simulink model "Template_v4_1_0_2024b_Jetson"  (R2024b)
settings: Solver=ode4  StartTime=0.0  StopTime=tsim  FixedStep=baseRate  RelTol=1e-6  AbsTol=1e-6
undefined symbols (not defined in the file): a1, a2, a3, b0, b1, b2, b3, baseRate, dataRate, DiscIntNeverNeededParam, drop_states_ARM, drop_states_BLACK, drop_states_BLUE, drop_states_RED, F_red_X_nominal, F_red_Y_nominal, F_thrusters_BLACK, F_thrusters_BLUE, F_thrusters_RED, Gamma1_el, Gamma1_sh, Gamma1_wr, Gamma2_el, Gamma2_sh, Gamma2_wr, Gamma3_el, Gamma3_sh, Gamma3_wr, Gamma4_el, Gamma4_sh, Gamma4_wr, Gamma5_el, Gamma5_sh, Gamma5_wr, Gamma6_el, Gamma6_sh, Gamma6_wr, home_states_BLACK, home_states_BLUE, home_states_RED, IBLACK, IBLUE, IDIST, IEE, init_states_BLACK, init_states_BLUE, init_states_RED, IPROX, IRED, K_BLACK, K_BLUE, K_RED, Kd_elarm, Kd_sharm, Kd_tb, Kd_tblue, Kd_tr, Kd_wrarm, Kd_xb, Kd_xblue ... (+45)
libraries: simulink x30, nvidiaSharedBlocks x19, MainLibrary x6, dspinverses x3, nvidiaIMUSensorslib x1
(part 6 of 8)

== system Template_v4_1_0_2024b_Jetson/1 - Experiment Logic/Phase #3: Experiment/Sub-Phase #3 /Desired Position BLUE/Wrap ==
  In1 : Inport
  Atan2 : Trigonometry  Operator=atan2
  Cos : Trigonometry  Operator=cos
  Sin : Trigonometry
  Out1 : Outport
  wires:
  In1/1 -> Sin/1, Cos/1
  Cos/1 -> Atan2/2
  Atan2/1 -> Out1/1
  Sin/1 -> Atan2/1

== system Template_v4_1_0_2024b_Jetson/1 - Experiment Logic/Phase #3: Experiment/Sub-Phase #3 /Desired Position RED/Calculate Circular Tracking ==
  Angular Frequency : Inport
  Constant1 : Constant  Value=xLength/2
  Constant2 : Constant  Value=yLength/2
  Cos : Trigonometry  Operator=cos
  Gain : Gain  Gain=0.85
  Gain1 : Gain  Gain=0.85
  Sin : Trigonometry
  Sum1 : Sum  Inputs=|++
  Sum2 : Sum  Inputs=|++
  Target X : Outport
  Target Y : Outport  Port=2
  wires:
  Constant2/1 -> Sum2/2
  Angular Frequency/1 -> Sin/1, Cos/1
  Constant1/1 -> Sum1/2
  Cos/1 -> Gain/1
  Gain1/1 -> Sum2/1
  Sin/1 -> Gain1/1
  Gain/1 -> Sum1/1
  Sum2/1 -> Target Y/1
  Sum1/1 -> Target X/1

== system Template_v4_1_0_2024b_Jetson/1 - Experiment Logic/Phase #3: Experiment/Sub-Phase #3 /Desired Position RED/Calculate Time since Phase #3 Start ==
  Constant2 : Constant  Value=Phase2_End  SampleTime=-1
  Subsystem : Subsystem
  Subtract3 : Sum  Inputs=+-
  Time : Outport  VectorParamsAs1DForOutWhenUnconnected=off
  wires:
  Subtract3/1 -> Time/1
  Constant2/1 -> Subtract3/2
  Subsystem/1(Time) -> Subtract3/1

== system Template_v4_1_0_2024b_Jetson/1 - Experiment Logic/Phase #3: Experiment/Sub-Phase #3 /Desired Position RED/Wrap ==
  In1 : Inport
  Atan2 : Trigonometry  Operator=atan2
  Cos : Trigonometry  Operator=cos
  Sin : Trigonometry
  Out1 : Outport
  wires:
  In1/1 -> Sin/1, Cos/1
  Cos/1 -> Atan2/2
  Atan2/1 -> Out1/1
  Sin/1 -> Atan2/1

== system Template_v4_1_0_2024b_Jetson/1 - Experiment Logic/Phase #3: Experiment/Sub-Phase #4/Desired Position BLACK/BLACK_Rz Desired ==
  Desired Rate (BLACK) : Constant  Value=0.03490659  SampleTime=-1
  Product : Product
  Subsystem : Subsystem
  Rz_Target : Outport  VectorParamsAs1DForOutWhenUnconnected=off
  wires:
  Product/1 -> Rz_Target/1
  Desired Rate (BLACK)/1 -> Product/1
  Subsystem/1(Time) -> Product/2

== system Template_v4_1_0_2024b_Jetson/1 - Experiment Logic/Phase #3: Experiment/Sub-Phase #4/Desired Position BLACK/Wrap ==
  In1 : Inport
  Atan2 : Trigonometry  Operator=atan2
  Cos : Trigonometry  Operator=cos
  Sin : Trigonometry
  Out1 : Outport
  wires:
  In1/1 -> Sin/1, Cos/1
  Cos/1 -> Atan2/2
  Atan2/1 -> Out1/1
  Sin/1 -> Atan2/1

== system Template_v4_1_0_2024b_Jetson/1 - Experiment Logic/Phase #3: Experiment/Sub-Phase #4/Desired Position BLUE/Calculate Circular Tracking ==
  Angular Frequency : Inport
  Constant1 : Constant  Value=xLength/2
  Constant2 : Constant  Value=yLength/2
  Cos : Trigonometry  Operator=cos
  Gain : Gain  Gain=-0.85
  Gain1 : Gain  Gain=-0.85
  Sin : Trigonometry
  Sum1 : Sum  Inputs=|++
  Sum2 : Sum  Inputs=|++
  Target X : Outport
  Target Y : Outport  Port=2
  wires:
  Constant2/1 -> Sum2/2
  Angular Frequency/1 -> Sin/1, Cos/1
  Constant1/1 -> Sum1/2
  Cos/1 -> Gain/1
  Gain1/1 -> Sum2/1
  Sin/1 -> Gain1/1
  Gain/1 -> Sum1/1
  Sum2/1 -> Target Y/1
  Sum1/1 -> Target X/1

== system Template_v4_1_0_2024b_Jetson/1 - Experiment Logic/Phase #3: Experiment/Sub-Phase #4/Desired Position BLUE/Calculate Time since Phase #3 Start ==
  Constant2 : Constant  Value=Phase2_End  SampleTime=-1
  Subsystem : Subsystem
  Subtract3 : Sum  Inputs=+-
  Time : Outport  VectorParamsAs1DForOutWhenUnconnected=off
  wires:
  Subtract3/1 -> Time/1
  Constant2/1 -> Subtract3/2
  Subsystem/1(Time) -> Subtract3/1

== system Template_v4_1_0_2024b_Jetson/1 - Experiment Logic/Phase #3: Experiment/Sub-Phase #4/Desired Position BLUE/Wrap ==
  In1 : Inport
  Atan2 : Trigonometry  Operator=atan2
  Cos : Trigonometry  Operator=cos
  Sin : Trigonometry
  Out1 : Outport
  wires:
  In1/1 -> Sin/1, Cos/1
  Cos/1 -> Atan2/2
  Atan2/1 -> Out1/1
  Sin/1 -> Atan2/1

== system Template_v4_1_0_2024b_Jetson/1 - Experiment Logic/Phase #3: Experiment/Sub-Phase #4/Desired Position RED/Calculate Circular Tracking ==
  Angular Frequency : Inport
  Constant1 : Constant  Value=xLength/2
  Constant2 : Constant  Value=yLength/2
  Cos : Trigonometry  Operator=cos
  Gain : Gain  Gain=0.85
  Gain1 : Gain  Gain=0.85
  Sin : Trigonometry
  Sum1 : Sum  Inputs=|++
  Sum2 : Sum  Inputs=|++
  Target X : Outport
  Target Y : Outport  Port=2
  wires:
  Constant2/1 -> Sum2/2
  Angular Frequency/1 -> Sin/1, Cos/1
  Constant1/1 -> Sum1/2
  Cos/1 -> Gain/1
  Gain1/1 -> Sum2/1
  Sin/1 -> Gain1/1
  Gain/1 -> Sum1/1
  Sum2/1 -> Target Y/1
  Sum1/1 -> Target X/1

== system Template_v4_1_0_2024b_Jetson/1 - Experiment Logic/Phase #3: Experiment/Sub-Phase #4/Desired Position RED/Calculate Time since Phase #3 Start ==
  Constant2 : Constant  Value=Phase2_End  SampleTime=-1
  Subsystem : Subsystem
  Subtract3 : Sum  Inputs=+-
  Time : Outport  VectorParamsAs1DForOutWhenUnconnected=off
  wires:
  Subtract3/1 -> Time/1
  Constant2/1 -> Subtract3/2
  Subsystem/1(Time) -> Subtract3/1

== system Template_v4_1_0_2024b_Jetson/1 - Experiment Logic/Phase #3: Experiment/Sub-Phase #4/Desired Position RED/Wrap ==
  In1 : Inport
  Atan2 : Trigonometry  Operator=atan2
  Cos : Trigonometry  Operator=cos
  Sin : Trigonometry
  Out1 : Outport
  wires:
  In1/1 -> Sin/1, Cos/1
  Cos/1 -> Atan2/2
  Atan2/1 -> Out1/1
  Sin/1 -> Atan2/1

== system Template_v4_1_0_2024b_Jetson/PhaseSpace Camera Code/Use Hardware to Obtain States/Receive and Process Phasespace Data/Check for Sychronization (Updated)/Enabled Subsystem2 ==
  In1 : Inport
  Enable : EnablePort
  Universal Time : Outport
  wires:
  In1/1 -> Universal Time/1

== system Template_v4_1_0_2024b_Jetson/PhaseSpace Camera Code/Use Hardware to Obtain States/Receive and Process Phasespace Data/Check for Sychronization (Updated)/Send Sync. Time ==
  Universal Time : Inport
  Change BLACK Behavior : Subsystem  TreatAsAtomicUnit=on
  Change BLUE Behavior : Subsystem  TreatAsAtomicUnit=on
  Change RED Behavior : Subsystem  TreatAsAtomicUnit=on
  Data Store Read : DataStoreRead  DataStoreName=WhoAmI  IndexOptions=Index vector (dialog)  Indices=1  OutputSizes=1
  Data Store Read2 : DataStoreRead  DataStoreName=isSim  IndexOptions=Index vector (dialog)  Indices=1  OutputSizes=1
  This IF block determines whether or not to run the BLACK sim/exp : If  NumInputs=2  IfExpression=u1 == 2 & u2 == 0  ShowElse=off
  This IF block determines whether or not to run the BLUE sim/exp : If  NumInputs=2  IfExpression=u1 == 3 & u2 == 0  ShowElse=off
  "This IF block determines whether or not to run the RED sim/exp " : If  NumInputs=2  IfExpression=u1 == 1 & u2 == 0  ShowElse=off
  wires:
  Data Store Read/1 -> This IF block determines whether or not to run the BLUE sim/exp/1, This IF block determines whether or not to run the BLACK sim/exp/1, "This IF block determines whether or not to run the RED sim/exp "/1
  This IF block determines whether or not to run the BLUE sim/exp/1 -> Change BLUE Behavior/Action
  "This IF block determines whether or not to run the RED sim/exp "/1 -> Change RED Behavior/Action
  Data Store Read2/1 -> This IF block determines whether or not to run the BLACK sim/exp/2, This IF block determines whether or not to run the BLUE sim/exp/2, "This IF block determines whether or not to run the RED sim/exp "/2
  This IF block determines whether or not to run the BLACK sim/exp/1 -> Change BLACK Behavior/Action
  Universal Time/1 -> Change BLACK Behavior/1(Universal Time), Change RED Behavior/1(Universal Time), Change BLUE Behavior/1(Universal Time)

== system Template_v4_1_0_2024b_Jetson/PhaseSpace Camera Code/Use Hardware to Obtain States/Store BLACK Data/Calculate True Time Step/Enabled Subsystem3 ==
  y2-y1 : Inport
  Enable : EnablePort
  dy(t)/dt : Outport
  wires:
  y2-y1/1 -> dy(t)/dt/1

== system Template_v4_1_0_2024b_Jetson/PhaseSpace Camera Code/Use Hardware to Obtain States/Store BLACK Data/Subsystem1/Enabled Subsystem ==
  y : Inport
  dt : Inport  Port=2
  Enable : EnablePort
  Constant2 : Constant  Value=0.1
  Delay : Delay  DelayLength=1
  MATLAB Function : MATLAB Function  TreatAsAtomicUnit=on
  dy/dt : Outport
  wires:
  Constant2/1 -> MATLAB Function/3(tau)
  dt/1 -> MATLAB Function/2(dt)
  Delay/1 -> MATLAB Function/4(ema_prev)
  MATLAB Function/2(ema) -> Delay/1
  y/1 -> MATLAB Function/1(y)
  MATLAB Function/1(dy) -> dy/dt/1

== system Template_v4_1_0_2024b_Jetson/PhaseSpace Camera Code/Use Hardware to Obtain States/Store BLACK Data/Subsystem2/Enabled Subsystem ==
  y : Inport
  dt : Inport  Port=2
  Enable : EnablePort
  Constant2 : Constant  Value=0.1
  Delay : Delay  DelayLength=1
  MATLAB Function : MATLAB Function  TreatAsAtomicUnit=on
  dy/dt : Outport
  wires:
  Constant2/1 -> MATLAB Function/3(tau)
  dt/1 -> MATLAB Function/2(dt)
  Delay/1 -> MATLAB Function/4(ema_prev)
  MATLAB Function/2(ema) -> Delay/1
  y/1 -> MATLAB Function/1(y)
  MATLAB Function/1(dy) -> dy/dt/1

== system Template_v4_1_0_2024b_Jetson/PhaseSpace Camera Code/Use Hardware to Obtain States/Store BLUE Data/Calculate True Time Step/Enabled Subsystem3 ==
  y2-y1 : Inport
  Enable : EnablePort
  dy(t)/dt : Outport
  wires:
  y2-y1/1 -> dy(t)/dt/1

== system Template_v4_1_0_2024b_Jetson/PhaseSpace Camera Code/Use Hardware to Obtain States/Store BLUE Data/Subsystem1/Enabled Subsystem ==
  y : Inport
  dt : Inport  Port=2
  Enable : EnablePort
  Constant2 : Constant  Value=0.1
  Delay : Delay  DelayLength=1
  MATLAB Function : MATLAB Function  TreatAsAtomicUnit=on
  dy/dt : Outport
  wires:
  Constant2/1 -> MATLAB Function/3(tau)
  dt/1 -> MATLAB Function/2(dt)
  Delay/1 -> MATLAB Function/4(ema_prev)
  MATLAB Function/2(ema) -> Delay/1
  y/1 -> MATLAB Function/1(y)
  MATLAB Function/1(dy) -> dy/dt/1

== system Template_v4_1_0_2024b_Jetson/PhaseSpace Camera Code/Use Hardware to Obtain States/Store BLUE Data/Subsystem2/Enabled Subsystem ==
  y : Inport
  dt : Inport  Port=2
  Enable : EnablePort
  Constant2 : Constant  Value=0.1
  Delay : Delay  DelayLength=1
  MATLAB Function : MATLAB Function  TreatAsAtomicUnit=on
  dy/dt : Outport
  wires:
  Constant2/1 -> MATLAB Function/3(tau)
  dt/1 -> MATLAB Function/2(dt)
  Delay/1 -> MATLAB Function/4(ema_prev)
  MATLAB Function/2(ema) -> Delay/1
  y/1 -> MATLAB Function/1(y)
  MATLAB Function/1(dy) -> dy/dt/1

== system Template_v4_1_0_2024b_Jetson/PhaseSpace Camera Code/Use Hardware to Obtain States/Store RED Data/Calculate True Time Step/Enabled Subsystem3 ==
  y2-y1 : Inport
  Enable : EnablePort
  dy(t)/dt : Outport
  wires:
  y2-y1/1 -> dy(t)/dt/1

== system Template_v4_1_0_2024b_Jetson/PhaseSpace Camera Code/Use Hardware to Obtain States/Store RED Data/Subsystem1/Enabled Subsystem ==
  y : Inport
  dt : Inport  Port=2
  Enable : EnablePort
  Constant2 : Constant  Value=0.1
  Delay : Delay  DelayLength=1
  MATLAB Function : MATLAB Function  TreatAsAtomicUnit=on
  dy/dt : Outport
  wires:
  Constant2/1 -> MATLAB Function/3(tau)
  dt/1 -> MATLAB Function/2(dt)
  Delay/1 -> MATLAB Function/4(ema_prev)
  MATLAB Function/2(ema) -> Delay/1
  y/1 -> MATLAB Function/1(y)
  MATLAB Function/1(dy) -> dy/dt/1

== system Template_v4_1_0_2024b_Jetson/PhaseSpace Camera Code/Use Hardware to Obtain States/Store RED Data/Subsystem2/Enabled Subsystem ==
  y : Inport
  dt : Inport  Port=2
  Enable : EnablePort
  Constant2 : Constant  Value=0.1
  Delay : Delay  DelayLength=1
  MATLAB Function : MATLAB Function  TreatAsAtomicUnit=on
  dy/dt : Outport
  wires:
  Constant2/1 -> MATLAB Function/3(tau)
  dt/1 -> MATLAB Function/2(dt)
  Delay/1 -> MATLAB Function/4(ema_prev)
  MATLAB Function/2(ema) -> Delay/1
  y/1 -> MATLAB Function/1(y)
  MATLAB Function/1(dy) -> dy/dt/1

== system Template_v4_1_0_2024b_Jetson/Simulate Plant Dynamics/BLACK Dynamics/Calculated & Store Measured States/Subsystem1/Enabled Subsystem ==
  y : Inport
  dt : Inport  Port=2
  Enable : EnablePort
  Constant2 : Constant  Value=0.1
  Delay : Delay  DelayLength=1
  MATLAB Function : MATLAB Function  TreatAsAtomicUnit=on
  dy/dt : Outport
  wires:
  Constant2/1 -> MATLAB Function/3(tau)
  dt/1 -> MATLAB Function/2(dt)
  Delay/1 -> MATLAB Function/4(ema_prev)
  MATLAB Function/2(ema) -> Delay/1
  y/1 -> MATLAB Function/1(y)
  MATLAB Function/1(dy) -> dy/dt/1

== system Template_v4_1_0_2024b_Jetson/Simulate Plant Dynamics/BLACK Dynamics/Calculated & Store Measured States/Subsystem2/Enabled Subsystem ==
  y : Inport
  dt : Inport  Port=2
  Enable : EnablePort
  Constant2 : Constant  Value=0.1
  Delay : Delay  DelayLength=1
  MATLAB Function : MATLAB Function  TreatAsAtomicUnit=on
  dy/dt : Outport
  wires:
  Constant2/1 -> MATLAB Function/3(tau)
  dt/1 -> MATLAB Function/2(dt)
  Delay/1 -> MATLAB Function/4(ema_prev)
  MATLAB Function/2(ema) -> Delay/1
  y/1 -> MATLAB Function/1(y)
  MATLAB Function/1(dy) -> dy/dt/1

== system Template_v4_1_0_2024b_Jetson/Simulate Plant Dynamics/BLACK Dynamics/Data @ Measurement Rate/Calculate True Time Step/Enabled Subsystem3 ==
  y2-y1 : Inport
  Enable : EnablePort
  dy(t)/dt : Outport
  wires:
  y2-y1/1 -> dy(t)/dt/1

== system Template_v4_1_0_2024b_Jetson/Simulate Plant Dynamics/BLUE Dynamics/Calculated & Store Measured States/Subsystem1/Enabled Subsystem ==
  y : Inport
  dt : Inport  Port=2
  Enable : EnablePort
  Constant2 : Constant  Value=0.1
  Delay : Delay  DelayLength=1
  MATLAB Function : MATLAB Function  TreatAsAtomicUnit=on
  dy/dt : Outport
  wires:
  Constant2/1 -> MATLAB Function/3(tau)
  dt/1 -> MATLAB Function/2(dt)
  Delay/1 -> MATLAB Function/4(ema_prev)
  MATLAB Function/2(ema) -> Delay/1
  y/1 -> MATLAB Function/1(y)
  MATLAB Function/1(dy) -> dy/dt/1

== system Template_v4_1_0_2024b_Jetson/Simulate Plant Dynamics/BLUE Dynamics/Calculated & Store Measured States/Subsystem2/Enabled Subsystem ==
  y : Inport
  dt : Inport  Port=2
  Enable : EnablePort
  Constant2 : Constant  Value=0.1
  Delay : Delay  DelayLength=1
  MATLAB Function : MATLAB Function  TreatAsAtomicUnit=on
  dy/dt : Outport
  wires:
  Constant2/1 -> MATLAB Function/3(tau)
  dt/1 -> MATLAB Function/2(dt)
  Delay/1 -> MATLAB Function/4(ema_prev)
  MATLAB Function/2(ema) -> Delay/1
  y/1 -> MATLAB Function/1(y)
  MATLAB Function/1(dy) -> dy/dt/1

== system Template_v4_1_0_2024b_Jetson/Simulate Plant Dynamics/BLUE Dynamics/Data @ Measurement Rate/Calculate True Time Step/Enabled Subsystem3 ==
  y2-y1 : Inport
  Enable : EnablePort
  dy(t)/dt : Outport
  wires:
  y2-y1/1 -> dy(t)/dt/1

== system Template_v4_1_0_2024b_Jetson/Simulate Plant Dynamics/RED and ARM Dynamics/RED + ARM/Calculated & Store Measured States/Subsystem3 ==
  dt : Inport
  y : Inport  Port=2
  Constant3 : Constant  Value=0
  Delay1 : Delay  DelayLength=1
  Enabled Subsystem : Subsystem  TreatAsAtomicUnit=on
  Relational Operator : RelationalOperator  Operator=~=  OutDataTypeStr=boolean  RndMeth=Simplest  InputSameDT=off
  Subtract1 : Sum  Inputs=+-
  dy/dt : Outport
  wires:
  Constant3/1 -> Relational Operator/2
  Relational Operator/1 -> Enabled Subsystem/Enable
  Delay1/1 -> Subtract1/2
  dt/1 -> Enabled Subsystem/2(dt)
  Subtract1/1 -> Relational Operator/1
  Enabled Subsystem/1(dy/dt) -> dy/dt/1
  y/1 -> Enabled Subsystem/1(y), Delay1/1, Subtract1/1

== system Template_v4_1_0_2024b_Jetson/Simulate Plant Dynamics/RED and ARM Dynamics/RED + ARM/Calculated & Store Measured States/Subsystem4 ==
  dt : Inport
  y : Inport  Port=2
  Constant3 : Constant  Value=0
  Delay1 : Delay  DelayLength=1
  Enabled Subsystem : Subsystem  TreatAsAtomicUnit=on
  Relational Operator : RelationalOperator  Operator=~=  OutDataTypeStr=boolean  RndMeth=Simplest  InputSameDT=off
  Subtract1 : Sum  Inputs=+-
  dy/dt : Outport
  wires:
  Constant3/1 -> Relational Operator/2
  Relational Operator/1 -> Enabled Subsystem/Enable
  Delay1/1 -> Subtract1/2
  dt/1 -> Enabled Subsystem/2(dt)
  Subtract1/1 -> Relational Operator/1
  Enabled Subsystem/1(dy/dt) -> dy/dt/1
  y/1 -> Enabled Subsystem/1(y), Delay1/1, Subtract1/1

== system Template_v4_1_0_2024b_Jetson/Simulate Plant Dynamics/RED and ARM Dynamics/RED + ARM/Calculated & Store Measured States/Subsystem5 ==
  dt : Inport
  y : Inport  Port=2
  Constant3 : Constant  Value=0
  Delay1 : Delay  DelayLength=1
  Enabled Subsystem : Subsystem  TreatAsAtomicUnit=on
  Relational Operator : RelationalOperator  Operator=~=  OutDataTypeStr=boolean  RndMeth=Simplest  InputSameDT=off
  Subtract1 : Sum  Inputs=+-
  dy/dt : Outport
  wires:
  Constant3/1 -> Relational Operator/2
  Relational Operator/1 -> Enabled Subsystem/Enable
  Delay1/1 -> Subtract1/2
  dt/1 -> Enabled Subsystem/2(dt)
  Subtract1/1 -> Relational Operator/1
  Enabled Subsystem/1(dy/dt) -> dy/dt/1
  y/1 -> Enabled Subsystem/1(y), Delay1/1, Subtract1/1

== system Template_v4_1_0_2024b_Jetson/Simulate Plant Dynamics/RED and ARM Dynamics/RED + ARM/Calculated & Store Measured States/Wrap ==
  Unwrapped Angle : Inport
  Atan2 : Trigonometry  Operator=atan2
  Cos : Trigonometry  Operator=cos
  Sin : Trigonometry
  Wrapped Angle : Outport
  wires:
  Unwrapped Angle/1 -> Sin/1, Cos/1
  Cos/1 -> Atan2/2
  Atan2/1 -> Wrapped Angle/1
  Sin/1 -> Atan2/1

== system Template_v4_1_0_2024b_Jetson/Simulate Plant Dynamics/RED and ARM Dynamics/RED + ARM/Calculated & Store True States/Wrap ==
  Unwrapped Angle : Inport
  Atan2 : Trigonometry  Operator=atan2
  Cos : Trigonometry  Operator=cos
  Sin : Trigonometry
  Wrapped Angle : Outport
  wires:
  Unwrapped Angle/1 -> Sin/1, Cos/1
  Cos/1 -> Atan2/2
  Atan2/1 -> Wrapped Angle/1
  Sin/1 -> Atan2/1

== system Template_v4_1_0_2024b_Jetson/Simulate Plant Dynamics/RED and ARM Dynamics/RED + ARM/Data @ Measurement Rate/Calculate True Time Step ==
  Data : Inport
  Time : Inport  Port=2
  Rate : Inport  Port=3
  Constant3 : Constant  Value=0
  Delay1 : Delay  DelayLength=1  InitialCondition=0
  Delay2 : Delay  DelayLength=1  InitialCondition=0
  Demux : Demux  Outputs=[1,5]
  Enabled Subsystem3 : Subsystem  TreatAsAtomicUnit=on
  MATLAB Function : MATLAB Function  TreatAsAtomicUnit=on
  Relational Operator : RelationalOperator  Operator=~=  OutDataTypeStr=boolean  RndMeth=Simplest  InputSameDT=off
  Subtract1 : Sum  Inputs=+-
  Subtract2 : Sum  Inputs=+-
  Terminator : Terminator
  dt_out : Outport
  wires:
  Rate/1 -> MATLAB Function/2(dataRate)
  MATLAB Function/1(dt_out) -> dt_out/1
  Time/1 -> Delay2/1, Subtract1/1
  Enabled Subsystem3/1(dy(t)/dt) -> MATLAB Function/1(dt)
  Data/1 -> Demux/1
  Subtract2/1 -> Relational Operator/1
  Relational Operator/1 -> Enabled Subsystem3/Enable
  Constant3/1 -> Relational Operator/2
  Demux/1 -> Subtract2/1, Delay1/1
  Delay1/1 -> Subtract2/2
  Demux/2 -> Terminator/1
  Subtract1/1 -> Enabled Subsystem3/1(y2-y1)
  Delay2/1 -> Subtract1/2

== system Template_v4_1_0_2024b_Jetson/Simulate Plant Dynamics/RED and ARM Dynamics/RED + ARM/Data @ Measurement Rate/Enabled Subsystem ==
  In1 : Inport
  Enable : EnablePort
  Out1 : Outport
  wires:
  In1/1 -> Out1/1

== system Template_v4_1_0_2024b_Jetson/Simulate Plant Dynamics/RED and ARM Dynamics/RED + ARM/Data @ Measurement Rate/Enabled Subsystem1 ==
  ThrustPer_Final : Inport
  Enable : EnablePort
  Out1 : Outport
  wires:
  ThrustPer_Final/1 -> Out1/1

== system Template_v4_1_0_2024b_Jetson/Simulate Plant Dynamics/RED and ARM Dynamics/RED Only/Calculated & Store Measured States/Subsystem1 ==
  dt : Inport
  y : Inport  Port=2
  Constant3 : Constant  Value=0
  Delay1 : Delay  DelayLength=1
  Enabled Subsystem : Subsystem  TreatAsAtomicUnit=on
  Relational Operator : RelationalOperator  Operator=~=  OutDataTypeStr=boolean  RndMeth=Simplest  InputSameDT=off
  Subtract1 : Sum  Inputs=+-
  dy/dt : Outport
  wires:
  Constant3/1 -> Relational Operator/2
  Relational Operator/1 -> Enabled Subsystem/Enable
  Delay1/1 -> Subtract1/2
  dt/1 -> Enabled Subsystem/2(dt)
  Subtract1/1 -> Relational Operator/1
  Enabled Subsystem/1(dy/dt) -> dy/dt/1
  y/1 -> Enabled Subsystem/1(y), Delay1/1, Subtract1/1

== system Template_v4_1_0_2024b_Jetson/Simulate Plant Dynamics/RED and ARM Dynamics/RED Only/Calculated & Store Measured States/Subsystem2 ==
  dt : Inport
  y : Inport  Port=2
  Constant3 : Constant  Value=0
  Delay1 : Delay  DelayLength=1
  Enabled Subsystem : Subsystem  TreatAsAtomicUnit=on
  Relational Operator : RelationalOperator  Operator=~=  OutDataTypeStr=boolean  RndMeth=Simplest  InputSameDT=off
  Subtract1 : Sum  Inputs=+-
  dy/dt : Outport
  wires:
  Constant3/1 -> Relational Operator/2
  Relational Operator/1 -> Enabled Subsystem/Enable
  Delay1/1 -> Subtract1/2
  dt/1 -> Enabled Subsystem/2(dt)
  Subtract1/1 -> Relational Operator/1
  Enabled Subsystem/1(dy/dt) -> dy/dt/1
  y/1 -> Delay1/1, Subtract1/1, Enabled Subsystem/1(y)

== system Template_v4_1_0_2024b_Jetson/Simulate Plant Dynamics/RED and ARM Dynamics/RED Only/Calculated & Store Measured States/Wrap ==
  Unwrapped Angle : Inport
  Atan2 : Trigonometry  Operator=atan2
  Cos : Trigonometry  Operator=cos
  Sin : Trigonometry
  Wrapped Angle : Outport
  wires:
  Unwrapped Angle/1 -> Sin/1, Cos/1
  Cos/1 -> Atan2/2
  Atan2/1 -> Wrapped Angle/1
  Sin/1 -> Atan2/1

== system Template_v4_1_0_2024b_Jetson/Simulate Plant Dynamics/RED and ARM Dynamics/RED Only/Calculated & Store True States/Wrap ==
  Unwrapped Angle : Inport
  Atan2 : Trigonometry  Operator=atan2
  Cos : Trigonometry  Operator=cos
  Sin : Trigonometry
  Wrapped Angle : Outport
  wires:
  Unwrapped Angle/1 -> Sin/1, Cos/1
  Cos/1 -> Atan2/2
  Atan2/1 -> Wrapped Angle/1
  Sin/1 -> Atan2/1

== system Template_v4_1_0_2024b_Jetson/Simulate Plant Dynamics/RED and ARM Dynamics/RED Only/Data @ Measurement Rate/Calculate True Time Step ==
  Data : Inport
  Time : Inport  Port=2
  Rate : Inport  Port=3
  Constant3 : Constant  Value=0
  Delay1 : Delay  DelayLength=1  InitialCondition=0
  Delay2 : Delay  DelayLength=1  InitialCondition=0
  Demux : Demux  Outputs=3
  Enabled Subsystem3 : Subsystem  TreatAsAtomicUnit=on
  MATLAB Function : MATLAB Function  TreatAsAtomicUnit=on
  Relational Operator : RelationalOperator  Operator=~=  OutDataTypeStr=boolean  RndMeth=Simplest  InputSameDT=off
  Subtract1 : Sum  Inputs=+-
  Subtract2 : Sum  Inputs=+-
  Terminator : Terminator
  Terminator1 : Terminator
  dt_out : Outport
  wires:
  Demux/3 -> Terminator1/1
  Rate/1 -> MATLAB Function/2(dataRate)
  MATLAB Function/1(dt_out) -> dt_out/1
  Time/1 -> Delay2/1, Subtract1/1
  Enabled Subsystem3/1(dy(t)/dt) -> MATLAB Function/1(dt)
  Data/1 -> Demux/1
  Subtract2/1 -> Relational Operator/1
  Relational Operator/1 -> Enabled Subsystem3/Enable
  Constant3/1 -> Relational Operator/2
  Demux/1 -> Subtract2/1, Delay1/1
  Delay1/1 -> Subtract2/2
  Demux/2 -> Terminator/1
  Subtract1/1 -> Enabled Subsystem3/1(y2-y1)
  Delay2/1 -> Subtract1/2

== system Template_v4_1_0_2024b_Jetson/Simulate Plant Dynamics/RED and ARM Dynamics/RED Only/Data @ Measurement Rate/Enabled Subsystem ==
  In1 : Inport
  Enable : EnablePort
  Out1 : Outport
  wires:
  In1/1 -> Out1/1

== system Template_v4_1_0_2024b_Jetson/Simulate Plant Dynamics/RED and ARM Dynamics/RED Only/Data @ Measurement Rate/Enabled Subsystem1 ==
  ThrustPer_Final : Inport
  Enable : EnablePort
  Out1 : Outport
  wires:
  ThrustPer_Final/1 -> Out1/1

== system Template_v4_1_0_2024b_Jetson/Thruster Control Code/Change BLACK Behavior/Calculate Duty Cycle/Duty Cycle @ PWM/Enabled Subsystem ==
  In1 : Inport
  Enable : EnablePort
  Out1 : Outport
  wires:
  In1/1 -> Out1/1

== system Template_v4_1_0_2024b_Jetson/Thruster Control Code/Change BLACK Behavior/Calculate Duty Cycle/Duty Cycle @ PWM/Enabled Subsystem1 ==
  ThrustPer_Final : Inport
  Enable : EnablePort
  Out1 : Outport
  wires:
  ThrustPer_Final/1 -> Out1/1

== system Template_v4_1_0_2024b_Jetson/Thruster Control Code/Change BLUE Behavior/Calculate Duty Cycle/Duty Cycle @ PWM/Enabled Subsystem ==
  In1 : Inport
  Enable : EnablePort
  Out1 : Outport
  wires:
  In1/1 -> Out1/1

== system Template_v4_1_0_2024b_Jetson/Thruster Control Code/Change BLUE Behavior/Calculate Duty Cycle/Duty Cycle @ PWM/Enabled Subsystem1 ==
  ThrustPer_Final : Inport
  Enable : EnablePort
  Out1 : Outport
  wires:
  ThrustPer_Final/1 -> Out1/1

== system Template_v4_1_0_2024b_Jetson/Thruster Control Code/Change RED Behavior/Calculate Duty Cycle/Duty Cycle @ PWM/Enabled Subsystem ==
  In1 : Inport
  Enable : EnablePort
  Out1 : Outport
  wires:
  In1/1 -> Out1/1

== system Template_v4_1_0_2024b_Jetson/Thruster Control Code/Change RED Behavior/Calculate Duty Cycle/Duty Cycle @ PWM/Enabled Subsystem1 ==
  ThrustPer_Final : Inport
  Enable : EnablePort
  Out1 : Outport
  wires:
  ThrustPer_Final/1 -> Out1/1

== system Template_v4_1_0_2024b_Jetson/1 - Experiment Logic/Phase #3: Experiment/Sub-Phase #1/Desired Position BLACK/BLACK_Rz Desired/Subsystem ==
  Constant1 : Constant  Value=Phase2_End  SampleTime=-1
  Subtract : Sum  Inputs=+-
  Universal_Time : DataStoreRead  DataStoreName=Univ_Time  IndexOptions=Index vector (dialog)  Indices=1  OutputSizes=1
  Time : Outport  VectorParamsAs1DForOutWhenUnconnected=off
  wires:
  Universal_Time/1 -> Subtract/1
  Subtract/1 -> Time/1
  Constant1/1 -> Subtract/2

== system Template_v4_1_0_2024b_Jetson/1 - Experiment Logic/Phase #3: Experiment/Sub-Phase #1/Desired Position BLUE/Calculate Time since Phase #3 Start/Subsystem ==
  Universal_Time : DataStoreRead  DataStoreName=Univ_Time  IndexOptions=Index vector (dialog)  Indices=1  OutputSizes=1
  Time : Outport  VectorParamsAs1DForOutWhenUnconnected=off
  wires:
  Universal_Time/1 -> Time/1

== system Template_v4_1_0_2024b_Jetson/1 - Experiment Logic/Phase #3: Experiment/Sub-Phase #1/Desired Position RED/Calculate Time since Phase #3 Start/Subsystem ==
  Universal_Time : DataStoreRead  DataStoreName=Univ_Time  IndexOptions=Index vector (dialog)  Indices=1  OutputSizes=1
  Time : Outport  VectorParamsAs1DForOutWhenUnconnected=off
  wires:
  Universal_Time/1 -> Time/1

== system Template_v4_1_0_2024b_Jetson/1 - Experiment Logic/Phase #3: Experiment/Sub-Phase #2 /Desired Position BLACK/BLACK_Rz Desired/Subsystem ==
  Constant1 : Constant  Value=Phase2_End  SampleTime=-1
  Subtract : Sum  Inputs=+-
  Universal_Time : DataStoreRead  DataStoreName=Univ_Time  IndexOptions=Index vector (dialog)  Indices=1  OutputSizes=1
  Time : Outport  VectorParamsAs1DForOutWhenUnconnected=off
  wires:
  Universal_Time/1 -> Subtract/1
  Subtract/1 -> Time/1
  Constant1/1 -> Subtract/2

== system Template_v4_1_0_2024b_Jetson/1 - Experiment Logic/Phase #3: Experiment/Sub-Phase #2 /Desired Position BLUE/Calculate Time since Phase #3 Start/Subsystem ==
  Universal_Time : DataStoreRead  DataStoreName=Univ_Time  IndexOptions=Index vector (dialog)  Indices=1  OutputSizes=1
  Time : Outport  VectorParamsAs1DForOutWhenUnconnected=off
  wires:
  Universal_Time/1 -> Time/1

== system Template_v4_1_0_2024b_Jetson/1 - Experiment Logic/Phase #3: Experiment/Sub-Phase #2 /Desired Position RED/Calculate Time since Phase #3 Start/Subsystem ==
  Universal_Time : DataStoreRead  DataStoreName=Univ_Time  IndexOptions=Index vector (dialog)  Indices=1  OutputSizes=1
  Time : Outport  VectorParamsAs1DForOutWhenUnconnected=off
  wires:
  Universal_Time/1 -> Time/1

== system Template_v4_1_0_2024b_Jetson/1 - Experiment Logic/Phase #3: Experiment/Sub-Phase #3 /Desired Position BLACK/BLACK_Rz Desired/Subsystem ==
  Constant1 : Constant  Value=Phase2_End  SampleTime=-1
  Subtract : Sum  Inputs=+-
  Universal_Time : DataStoreRead  DataStoreName=Univ_Time  IndexOptions=Index vector (dialog)  Indices=1  OutputSizes=1
  Time : Outport  VectorParamsAs1DForOutWhenUnconnected=off
  wires:
  Universal_Time/1 -> Subtract/1
  Subtract/1 -> Time/1
  Constant1/1 -> Subtract/2

== system Template_v4_1_0_2024b_Jetson/1 - Experiment Logic/Phase #3: Experiment/Sub-Phase #3 /Desired Position BLUE/Calculate Time since Phase #3 Start/Subsystem ==
  Universal_Time : DataStoreRead  DataStoreName=Univ_Time  IndexOptions=Index vector (dialog)  Indices=1  OutputSizes=1
  Time : Outport  VectorParamsAs1DForOutWhenUnconnected=off
  wires:
  Universal_Time/1 -> Time/1

== system Template_v4_1_0_2024b_Jetson/1 - Experiment Logic/Phase #3: Experiment/Sub-Phase #3 /Desired Position RED/Calculate Time since Phase #3 Start/Subsystem ==
  Universal_Time : DataStoreRead  DataStoreName=Univ_Time  IndexOptions=Index vector (dialog)  Indices=1  OutputSizes=1
  Time : Outport  VectorParamsAs1DForOutWhenUnconnected=off
  wires:
  Universal_Time/1 -> Time/1

== system Template_v4_1_0_2024b_Jetson/1 - Experiment Logic/Phase #3: Experiment/Sub-Phase #4/Desired Position BLACK/BLACK_Rz Desired/Subsystem ==
  Constant1 : Constant  Value=Phase2_End  SampleTime=-1
  Subtract : Sum  Inputs=+-
  Universal_Time : DataStoreRead  DataStoreName=Univ_Time  IndexOptions=Index vector (dialog)  Indices=1  OutputSizes=1
  Time : Outport  VectorParamsAs1DForOutWhenUnconnected=off
  wires:
  Universal_Time/1 -> Subtract/1
  Subtract/1 -> Time/1
  Constant1/1 -> Subtract/2

== system Template_v4_1_0_2024b_Jetson/1 - Experiment Logic/Phase #3: Experiment/Sub-Phase #4/Desired Position BLUE/Calculate Time since Phase #3 Start/Subsystem ==
  Universal_Time : DataStoreRead  DataStoreName=Univ_Time  IndexOptions=Index vector (dialog)  Indices=1  OutputSizes=1
  Time : Outport  VectorParamsAs1DForOutWhenUnconnected=off
  wires:
  Universal_Time/1 -> Time/1

== system Template_v4_1_0_2024b_Jetson/1 - Experiment Logic/Phase #3: Experiment/Sub-Phase #4/Desired Position RED/Calculate Time since Phase #3 Start/Subsystem ==
  Universal_Time : DataStoreRead  DataStoreName=Univ_Time  IndexOptions=Index vector (dialog)  Indices=1  OutputSizes=1
  Time : Outport  VectorParamsAs1DForOutWhenUnconnected=off
  wires:
  Universal_Time/1 -> Time/1

== system Template_v4_1_0_2024b_Jetson/PhaseSpace Camera Code/Use Hardware to Obtain States/Receive and Process Phasespace Data/Check for Sychronization (Updated)/Send Sync. Time/Change BLACK Behavior ==
  Universal Time : Inport
  Action Port : ActionPort  ActionPortLabel=if(u1 == 2 & u2 == 0)
  UDP Send (GUI) : nvidiaSharedBlocks/UDP Send  remoteURL='255.255.255.255'  remotePort=48721  localURL='0.0.0.0'  localPortSource=Automatically determine  localPort=-1  sampletime=-1  blockPlatform=NVIDIA  separateLengthPort=0
      settings: LibrarySourceBlock=nvidiaNetworklib/UDP Send
  wires:
  Universal Time/1 -> UDP Send (GUI)/1

== system Template_v4_1_0_2024b_Jetson/PhaseSpace Camera Code/Use Hardware to Obtain States/Receive and Process Phasespace Data/Check for Sychronization (Updated)/Send Sync. Time/Change BLUE Behavior ==
  Universal Time : Inport
  Action Port : ActionPort  ActionPortLabel=if(u1 == 3 & u2 == 0)
  UDP Send (GUI) : nvidiaSharedBlocks/UDP Send  remoteURL='255.255.255.255'  remotePort=48722  localURL='0.0.0.0'  localPortSource=Automatically determine  localPort=-1  sampletime=-1  blockPlatform=NVIDIA  separateLengthPort=0
      settings: LibrarySourceBlock=nvidiaNetworklib/UDP Send
  wires:
  Universal Time/1 -> UDP Send (GUI)/1

== system Template_v4_1_0_2024b_Jetson/PhaseSpace Camera Code/Use Hardware to Obtain States/Receive and Process Phasespace Data/Check for Sychronization (Updated)/Send Sync. Time/Change RED Behavior ==
  Universal Time : Inport
  Action Port : ActionPort  ActionPortLabel=if(u1 == 1 & u2 == 0)
  UDP Send (GUI) : nvidiaSharedBlocks/UDP Send  remoteURL='255.255.255.255'  remotePort=48720  localURL='0.0.0.0'  localPortSource=Automatically determine  localPort=-1  sampletime=-1  blockPlatform=NVIDIA  separateLengthPort=0
      settings: LibrarySourceBlock=nvidiaNetworklib/UDP Send
  wires:
  Universal Time/1 -> UDP Send (GUI)/1

== system Template_v4_1_0_2024b_Jetson/Simulate Plant Dynamics/RED and ARM Dynamics/RED + ARM/Calculated & Store Measured States/Subsystem3/Enabled Subsystem ==
  y : Inport
  dt : Inport  Port=2
  Enable : EnablePort
  Constant2 : Constant  Value=0.1
  Delay : Delay  DelayLength=1
  MATLAB Function : MATLAB Function  TreatAsAtomicUnit=on
  dy/dt : Outport
  wires:
  Constant2/1 -> MATLAB Function/3(tau)
  dt/1 -> MATLAB Function/2(dt)
  Delay/1 -> MATLAB Function/4(ema_prev)
  MATLAB Function/2(ema) -> Delay/1
  y/1 -> MATLAB Function/1(y)
  MATLAB Function/1(dy) -> dy/dt/1

== system Template_v4_1_0_2024b_Jetson/Simulate Plant Dynamics/RED and ARM Dynamics/RED + ARM/Calculated & Store Measured States/Subsystem4/Enabled Subsystem ==
  y : Inport
  dt : Inport  Port=2
  Enable : EnablePort
  Constant2 : Constant  Value=0.1
  Delay : Delay  DelayLength=1
  MATLAB Function : MATLAB Function  TreatAsAtomicUnit=on
  dy/dt : Outport
  wires:
  Constant2/1 -> MATLAB Function/3(tau)
  dt/1 -> MATLAB Function/2(dt)
  Delay/1 -> MATLAB Function/4(ema_prev)
  MATLAB Function/2(ema) -> Delay/1
  y/1 -> MATLAB Function/1(y)
  MATLAB Function/1(dy) -> dy/dt/1

== system Template_v4_1_0_2024b_Jetson/Simulate Plant Dynamics/RED and ARM Dynamics/RED + ARM/Calculated & Store Measured States/Subsystem5/Enabled Subsystem ==
  y : Inport
  dt : Inport  Port=2
  Enable : EnablePort
  Constant2 : Constant  Value=0.1
  Delay : Delay  DelayLength=1
  MATLAB Function : MATLAB Function  TreatAsAtomicUnit=on
  dy/dt : Outport
  wires:
  Constant2/1 -> MATLAB Function/3(tau)
  dt/1 -> MATLAB Function/2(dt)
  Delay/1 -> MATLAB Function/4(ema_prev)
  MATLAB Function/2(ema) -> Delay/1
  y/1 -> MATLAB Function/1(y)
  MATLAB Function/1(dy) -> dy/dt/1

== system Template_v4_1_0_2024b_Jetson/Simulate Plant Dynamics/RED and ARM Dynamics/RED + ARM/Data @ Measurement Rate/Calculate True Time Step/Enabled Subsystem3 ==
  y2-y1 : Inport
  Enable : EnablePort
  dy(t)/dt : Outport
  wires:
  y2-y1/1 -> dy(t)/dt/1

== system Template_v4_1_0_2024b_Jetson/Simulate Plant Dynamics/RED and ARM Dynamics/RED Only/Calculated & Store Measured States/Subsystem1/Enabled Subsystem ==
  y : Inport
  dt : Inport  Port=2
  Enable : EnablePort
  Constant2 : Constant  Value=0.1
  Delay : Delay  DelayLength=1
  MATLAB Function : MATLAB Function  TreatAsAtomicUnit=on
  dy/dt : Outport
  wires:
  Constant2/1 -> MATLAB Function/3(tau)
  dt/1 -> MATLAB Function/2(dt)
  Delay/1 -> MATLAB Function/4(ema_prev)
  MATLAB Function/2(ema) -> Delay/1
  y/1 -> MATLAB Function/1(y)
  MATLAB Function/1(dy) -> dy/dt/1

== system Template_v4_1_0_2024b_Jetson/Simulate Plant Dynamics/RED and ARM Dynamics/RED Only/Calculated & Store Measured States/Subsystem2/Enabled Subsystem ==
  y : Inport
  dt : Inport  Port=2
  Enable : EnablePort
  Constant2 : Constant  Value=0.1
  Delay : Delay  DelayLength=1
  MATLAB Function : MATLAB Function  TreatAsAtomicUnit=on
  dy/dt : Outport
  wires:
  Constant2/1 -> MATLAB Function/3(tau)
  dt/1 -> MATLAB Function/2(dt)
  Delay/1 -> MATLAB Function/4(ema_prev)
  MATLAB Function/2(ema) -> Delay/1
  y/1 -> MATLAB Function/1(y)
  MATLAB Function/1(dy) -> dy/dt/1

== system Template_v4_1_0_2024b_Jetson/Simulate Plant Dynamics/RED and ARM Dynamics/RED Only/Data @ Measurement Rate/Calculate True Time Step/Enabled Subsystem3 ==
  y2-y1 : Inport
  Enable : EnablePort
  dy(t)/dt : Outport
  wires:
  y2-y1/1 -> dy(t)/dt/1

== matlab function Template_v4_1_0_2024b_Jetson/3 - Control/Default LQR Control (BLUE)/Calculate Error/MATLAB Function ==
  data: Rz_path input; Rz_error output; Rz_measured input
function Rz_error = SmoothAngularDifference(Rz_path, Rz_measured)

    Rz_error = mod(Rz_measured-Rz_path+pi, 2*pi)-pi;


end

== matlab function Template_v4_1_0_2024b_Jetson/3 - Control/Default PD Control (BLUE)/Calculate Error/MATLAB Function ==
  data: Rz_path input; Rz_error output; Rz_measured input
function Rz_error = SmoothAngularDifference(Rz_path, Rz_measured)

    Rz_error = mod(Rz_measured-Rz_path+pi, 2*pi)-pi;


end

== matlab function Template_v4_1_0_2024b_Jetson/Simulate Plant Dynamics/RED and ARM Dynamics/RED + ARM/Calculated & Store Measured States/Subsystem3/Enabled Subsystem/MATLAB Function ==
  data: y input; dy output; dt input; tau input; ema_prev input; ema output
function [dy, ema] = realtime_derivative_ema(y, dt, tau, ema_prev)
    % Compute smoothed derivative using Exponential Moving Average
    %
    % Inputs:
    %   y        : Current measurement
    %   dt       : Time step
    %   tau      : Time constant for EMA filter (larger = more smoothing)
    %   ema_prev : Previous EMA value
    %
    % Outputs:
    %   dy  : Smoothed derivative estimate
    %   ema : Updated EMA value
    
    % Calculate smoothing factor from time constant
    alpha = 1 - exp(-dt ./ tau);
    
    % Update Exponential Moving Average
    ema = alpha .* y + (1 - alpha) .* ema_prev;
    
    % Compute derivative using finite difference on smoothed values
    dy = (ema - ema_prev) ./ dt;
end

== matlab function Template_v4_1_0_2024b_Jetson/Simulate Plant Dynamics/RED and ARM Dynamics/RED Only/Calculated & Store Measured States/Subsystem2/Enabled Subsystem/MATLAB Function ==
  data: y input; dy output; dt input; tau input; ema_prev input; ema output
function [dy, ema] = realtime_derivative_ema(y, dt, tau, ema_prev)
    % Compute smoothed derivative using Exponential Moving Average
    %
    % Inputs:
    %   y        : Current measurement
    %   dt       : Time step
    %   tau      : Time constant for EMA filter (larger = more smoothing)
    %   ema_prev : Previous EMA value
    %
    % Outputs:
    %   dy  : Smoothed derivative estimate
    %   ema : Updated EMA value
    
    % Calculate smoothing factor from time constant
    alpha = 1 - exp(-dt ./ tau);
    
    % Update Exponential Moving Average
    ema = alpha .* y + (1 - alpha) .* ema_prev;
    
    % Compute derivative using finite difference on smoothed values
    dy = (ema - ema_prev) ./ dt;
end

== matlab function Template_v4_1_0_2024b_Jetson/Simulate Plant Dynamics/BLACK Dynamics/Calculated & Store Measured States/Subsystem1/Enabled Subsystem/MATLAB Function ==
  data: y input; dy output; dt input; tau input; ema_prev input; ema output
function [dy, ema] = realtime_derivative_ema(y, dt, tau, ema_prev)
    % Compute smoothed derivative using Exponential Moving Average
    %
    % Inputs:
    %   y        : Current measurement
    %   dt       : Time step
    %   tau      : Time constant for EMA filter (larger = more smoothing)
    %   ema_prev : Previous EMA value
    %
    % Outputs:
    %   dy  : Smoothed derivative estimate
    %   ema : Updated EMA value
    
    % Calculate smoothing factor from time constant
    alpha = 1 - exp(-dt ./ tau);
    
    % Update Exponential Moving Average
    ema = alpha .* y + (1 - alpha) .* ema_prev;
    
    % Compute derivative using finite difference on smoothed values
    dy = (ema - ema_prev) ./ dt;
end

== matlab function Template_v4_1_0_2024b_Jetson/Simulate Plant Dynamics/RED and ARM Dynamics/RED Only/Data @ Measurement Rate/Calculate True Time Step/MATLAB Function ==
  data: dt input; dt_out output; dataRate input
function dt_out = CheckforInvalidTime(dt, dataRate)

    if dt <= 0

        dt_out = dataRate;

    else

        dt_out = dt;

    end


end

== matlab function Template_v4_1_0_2024b_Jetson/Thruster Control Code/Change BLACK Behavior/Calculate Duty Cycle/MATLAB Function5 ==
  data: H_final output; u_desired input; duty_cycles output; x0 input; thruster_dist2CG_RED parameter; F_red_X_nominal parameter; F_red_Y_nominal parameter; max_iters parameter; tol parameter
function [H_final, duty_cycles] = optimize_duty_cycle_with_decay( ...
    u_desired, x0, thruster_dist2CG_RED, F_red_X_nominal, F_red_Y_nominal, max_iters, tol)
    %OPTIMIZE_DUTY_CYCLE_WITH_DECAY 
    %   Iteratively optimizes thruster duty cycles while updating thrust decay.
    %
    %   Inputs:
    %       u_desired           - Desired force/torque vector [Fx; Fy; M] (3x1)
    %       x0                  - Initial guess for duty cycles (8x1)
    %       thruster_dist2CG_RED- Distances of thrusters from CG (vector, mm)
    %       F_red_X_nominal     - Nominal X-direction thruster force (scalar, N)
    %       F_red_Y_nominal     - Nominal Y-direction thruster force (scalar, N)
    %       max_iters           - Maximum optimization iterations
    %       tol                 - Convergence tolerance (on duty cycles)
    %
    %   Outputs:
    %       H_final     - Final H-matrix including thrust decay (3x8)
    %       duty_cycles - Optimized duty cycles (8x1)
    %

    % ---------------------------
    % Initialization
    % ---------------------------
    num_thrusters      = length(x0); %#ok<NASGU> % reserved if needed later
    duty_cycles        = x0;                     % current solution
    thrust_decay_factor = 1;                     % initial decay
    prev_duty_cycles   = duty_cycles + 2*tol;    % force first iteration

    % ---------------------------
    % Iterative optimization
    % ---------------------------
    for iter = 1:max_iters
        % Build system matrix H with current decay factor
        H = MakeHWithDecay(thruster_dist2CG_RED, F_red_X_nominal, ...
                           thrust_decay_factor, F_red_Y_nominal);

        % Solve constrained least squares (box constraints: 0 ≤ x ≤ 1)
        duty_cycles = custom_constrained_least_squares(H, u_desired, duty_cycles);

        % Update decay factor based on the current duty cycles
        [thrust_decay_factor, ~] = check_thrust_decay(duty_cycles);

        % Check convergence (∞-norm difference)
        if norm(duty_cycles - prev_duty_cycles, Inf) < tol
            H_final = MakeHWithDecayRecalculateForce(thruster_dist2CG_RED, ...
                        F_red_X_nominal, thrust_decay_factor, F_red_Y_nominal);
            return;
        end

        % Update reference for next iteration
        prev_duty_cycles = duty_cycles;
    end

    % If not converged within max_iters, return final H with last decay
    H_final = MakeHWithDecayRecalculateForce(thruster_dist2CG_RED, ...
                F_red_X_nominal, thrust_decay_factor, F_red_Y_nominal);
end


% ========================================================================
% Custom Constrained Least Squares Solver
% ========================================================================
function x_opt = custom_constrained_least_squares(H, b, x0)
    %CUSTOM_CONSTRAINED_LEAST_SQUARES
    %   Solves min_x ||H*x - b||^2 subject to 0 <= x <= 1
    %   using projected gradient descent with backtracking line search.
    %
    %   Inputs:
    %       H   - System matrix (3x8)
    %       b   - Desired vector (3x1)
    %       x0  - Initial guess (8x1)
    %
    %   Output:
    %       x_opt - Optimal duty cycle vector (8x1)

    % Parameters
    max_iterations = 100;
    tolerance      = 1e-6;
    alpha          = 0.01;  % initial step size
    beta           = 0.5;   % backtracking factor

    % Initialization
    x      = x0;
    x_prev = x0 + 2*tolerance;

    % Precompute matrices
    HtH = H' * H;
    Htb = H' * b;

    for iter = 1:max_iterations
        % Gradient of ||H*x - b||^2
        gradient = 2 * (HtH*x - Htb);

        % Store objective for comparison
        current_obj = norm(H*x - b)^2;

        % Backtracking line search
        step_size = alpha;
        for ls_iter = 1:20
            x_new = x - step_size * gradient;
            x_new = max(0, min(1, x_new)); % project into [0,1]

            new_obj = norm(H*x_new - b)^2;
            if new_obj < current_obj
                break; % accept step
            else
                step_size = step_size * beta;
            end
        end

        % Update
        x = x_new;

        % Convergence check
        if norm(x - x_prev) < tolerance
            break;
        end

        % Adaptive step size tuning
        if iter > 1 && new_obj < current_obj
            alpha = min(alpha * 1.1, 0.1); % speed up if progress
        else
            alpha = alpha * 0.9;           % slow down otherwise
        end

        % Store for next iteration
        x_prev = x;
    end

    x_opt = x;
end


% ========================================================================
% Construct H-matrix (with decay factor)
% ========================================================================
function H = MakeHWithDecay(thruster_dist2CG, F_X_nominal, thrust_decay_factor, F_Y_nominal)
    %MAKEHWITHDECAY
    %   Builds the H matrix that maps thruster duty cycles to [Fx; Fy; M],
    %   applying thrust decay.
    %
    %   Outputs H as (3x8)

    % Convert thruster arm distances to meters
    adjusted_dist = thruster_dist2CG / 1000;

    % Thruster directions (X, Y, and moment arm)
    Vec1 = [-1; -1;  0;  0;  1;  1;  0;  0]; % X
    Vec2 = [ 0;  0;  1;  1;  0;  0; -1; -1]; % Y
    Vec3 = adjusted_dist;                    % moment (Z)

    Mat1 = [Vec1, Vec2, Vec3]';

    % Thruster forces (scaled by decay)
    F_thrusters = [F_X_nominal; F_X_nominal; ...
                   F_Y_nominal; F_Y_nominal; ...
                   F_X_nominal; F_X_nominal; ...
                   F_Y_nominal; F_Y_nominal] * thrust_decay_factor;

    % Build diagonal scaling
    Mat2 = diag(F_thrusters / 2);

    % Final mapping
    H = Mat1 * Mat2;
end


% ========================================================================
% Construct H-matrix (recalculate full force with decay)
% ========================================================================
function H = MakeHWithDecayRecalculateForce(thruster_dist2CG, F_X_nominal, thrust_decay_factor, F_Y_nominal)
    %MAKEHWITHDECAYRECALCULATEFORCE
    %   Same as MakeHWithDecay but applies full nominal force scaling.

    adjusted_dist = thruster_dist2CG / 1000;

    Vec1 = [-1; -1;  0;  0;  1;  1;  0;  0];
    Vec2 = [ 0;  0;  1;  1;  0;  0; -1; -1];
    Vec3 = adjusted_dist;

    Mat1 = [Vec1, Vec2, Vec3]';

    F_thrusters = [F_X_nominal; F_X_nominal; ...
                   F_Y_nominal; F_Y_nominal; ...
                   F_X_nominal; F_X_nominal; ...
                   F_Y_nominal; F_Y_nominal] * thrust_decay_factor;

    Mat2 = diag(F_thrusters);

    H = Mat1 * Mat2;
end


% ========================================================================
% Thrust Decay Update Rule
% ========================================================================
function [thrust_decay_factor, count] = check_thrust_decay(PWMs)
    %CHECK_THRUST_DECAY
    %   Updates thrust decay factor based on average duty cycle.
    %
    %   Inputs:
    %       PWMs - Duty cycle vector (8x1)
    %
    %   Outputs:
    %       thrust_decay_factor - Adjusted decay factor (scalar)
    %       count               - Number of active thrusters

    % Normalize if needed
    if max(PWMs) > 1
        PWMs = PWMs / max(PWMs);
    end
    
    % Active thrusters
    count = sum(PWMs > 0);
    
    % Mean duty cycle (only active thrusters)
    avg_duty = sum(max(PWMs, 0)) / max(count, 1);
    
    % Update rule (piecewise)
    if avg_duty < 0.3 || count == 0
        thrust_decay_factor = 1;
    else
        thrust_decay_factor = max(0.6 - 2*avg_duty + 1, 0.5);
    end
end

== matlab function Template_v4_1_0_2024b_Jetson/Simulate Plant Dynamics/RED and ARM Dynamics/RED + ARM/Calculated & Store Measured States/Subsystem4/Enabled Subsystem/MATLAB Function ==
  data: y input; dy output; dt input; tau input; ema_prev input; ema output
function [dy, ema] = realtime_derivative_ema(y, dt, tau, ema_prev)
    % Compute smoothed derivative using Exponential Moving Average
    %
    % Inputs:
    %   y        : Current measurement
    %   dt       : Time step
    %   tau      : Time constant for EMA filter (larger = more smoothing)
    %   ema_prev : Previous EMA value
    %
    % Outputs:
    %   dy  : Smoothed derivative estimate
    %   ema : Updated EMA value
    
    % Calculate smoothing factor from time constant
    alpha = 1 - exp(-dt ./ tau);
    
    % Update Exponential Moving Average
    ema = alpha .* y + (1 - alpha) .* ema_prev;
    
    % Compute derivative using finite difference on smoothed values
    dy = (ema - ema_prev) ./ dt;
end

== matlab function Template_v4_1_0_2024b_Jetson/PhaseSpace Camera Code/Use Hardware to Obtain States/Store RED Data/Subsystem1/Enabled Subsystem/MATLAB Function ==
  data: y input; dy output; dt input; tau input; ema_prev input; ema output
function [dy, ema] = realtime_derivative_ema(y, dt, tau, ema_prev)
    % Compute smoothed derivative using Exponential Moving Average
    %
    % Inputs:
    %   y        : Current measurement
    %   dt       : Time step
    %   tau      : Time constant for EMA filter (larger = more smoothing)
    %   ema_prev : Previous EMA value
    %
    % Outputs:
    %   dy  : Smoothed derivative estimate
    %   ema : Updated EMA value
    
    % Calculate smoothing factor from time constant
    alpha = 1 - exp(-dt ./ tau);
    
    % Update Exponential Moving Average
    ema = alpha .* y + (1 - alpha) .* ema_prev;
    
    % Compute derivative using finite difference on smoothed values
    dy = (ema - ema_prev) ./ dt;
end
